simulink model "ALL"  (R2018b)
settings: Solver=ode4  StartTime=12.1169  StopTime=12.2369  FixedStep=0.01/44100  RelTol=1e-3
libraries: dsparch4 x2, commsynccomp2 x2
settings Model: Creator=HsuWeiChe  LastModifiedBy=yangq

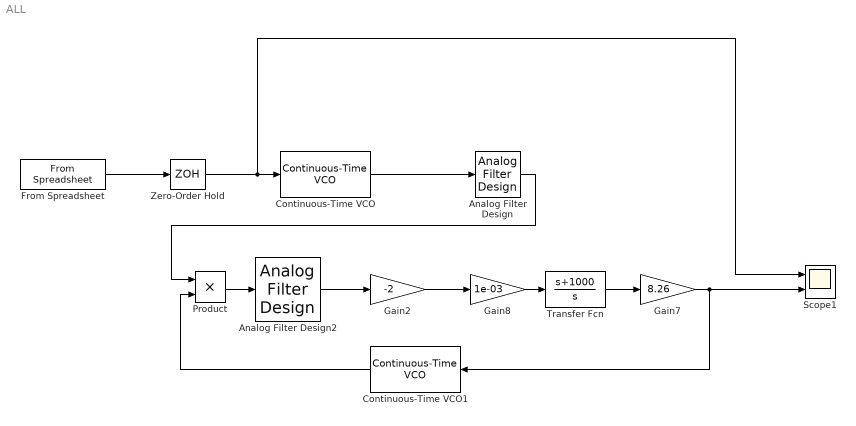
== system ALL ==
  Analog Filter Design : dsparch4/Analog Filter Design  method=Elliptic  filttype=Bandpass  N=6  Wlo=2*pi*(1e06-75000)  Whi=2*pi*(1e06+75000)  Rp=0.1  Rs=100
  Analog Filter Design2 : dsparch4/Analog Filter Design  method=Butterworth  filttype=Lowpass  N=6  Wlo=2*pi*22050  Whi=2*pi*(10^6+97050)  Rp=0.1  Rs=80
  Continuous-Time VCO : commsynccomp2/Continuous-Time VCO  Ac=1  Fc=1e06  Kc=77017  Ph=0
      settings: SourceProductName=Communications System Toolbox  SourceProductBaseCode=CM
  Continuous-Time VCO1 : commsynccomp2/Continuous-Time VCO  Ac=1  Fc=1e06  Kc=77017  Ph=-pi/2
      settings: SourceProductName=Communications System Toolbox  SourceProductBaseCode=CM
  From Spreadsheet : FromSpreadsheet  FileName=audio.xlsx  TreatFirstColumnAs=Data  SampleTime=-1
  Gain2 : Gain  Gain=-2
  Gain7 : Gain  Gain=8.26
  Gain8 : Gain  Gain=1e-03
  Product : Product
  Scope1 : Scope  NumInputPorts=2
  Transfer Fcn : TransferFcn  Numerator=[1 1000]  Denominator=[1 0]
  Zero-Order Hold : ZeroOrderHold  SampleTime=0.1/44100
  wires:
  Analog Filter Design/1 -> Product/1
  From Spreadsheet/1 -> Zero-Order Hold/1
  Zero-Order Hold/1 -> Scope1/1, Continuous-Time VCO/1
  Product/1 -> Analog Filter Design2/1
  Gain8/1 -> Transfer Fcn/1
  Transfer Fcn/1 -> Gain7/1
  Gain2/1 -> Gain8/1
  Analog Filter Design2/1 -> Gain2/1
  Continuous-Time VCO1/1 -> Product/2
  Gain7/1 -> Scope1/2, Continuous-Time VCO1/1
  Continuous-Time VCO/1 -> Analog Filter Design/1
